simulink library "thc"  (R2021b)
settings: Solver=VariableStepAuto  StartTime=0.0  StopTime=10.0  RelTol=1e-3
undefined symbols (not defined in the file or in its folder): ATHC_APTCQA_X_C, ATHC_APTCQB_X_C, ATHC_dAy_X_C, ATHC_Qeq_X_kmh, ATHC_VbaseC_X_C, ATHC_VbaseC_Y_W, ATHC_VbaseD_X_C, ATHC_VbaseH_X_C, FALSE, KTHC_ACMaxMinT_sec, KTHC_aDeice_K, KTHC_AGSDefLv_K, KTHC_AGSLv1_K, KTHC_AGSLv2_K, KTHC_AGSLv3_K, KTHC_AGSLv4_K, KTHC_AGSLv5_K, KTHC_AirIntUpdateT_sec, KTHC_APTCOneZoneMax_W, KTHC_APTCPeriod_cnt, KTHC_APTCPWMEN_flg, KTHC_APTCQMaxC_W, KTHC_APTCQminC_W, KTHC_APTCQminD_W, KTHC_APTCQminRe1_W, KTHC_APTCQminRe_W, KTHC_APTCQoffT_cnt, KTHC_APTCQonT_cnt, KTHC_APTCRiLeMaxDff_W, KTHC_APTCRiLeMinDff_W, KTHC_BatInTempDef_C, KTHC_bDeice_K, KTHC_CompMaxDeice_rpm, KTHC_CompMinDeice_rpm, KTHC_CompSotxvOp_K, KTHC_CompSotxvOpLow_rpm, KTHC_CompSpdmax_rpm, KTHC_CompSpdmaxBC1_rpm, KTHC_CompSpdmaxBC_rpm, KTHC_CompSpdmid1_rpm, KTHC_CompSpdmid2_rpm, KTHC_CompSpdmid3_rpm, KTHC_CompSpdmid_rpm, KTHC_CompSpdmin_rpm, KTHC_DAPTCQ1_W, KTHC_DAPTCQ2_W, KTHC_DAPTCQ3_W, KTHC_DcChSetTemp_C, KTHC_DehumidityEN_flg, KTHC_DeiceCycTime_K, KTHC_DriveLevelWPTCBAH1_W, KTHC_DriveLevelWPTCBAH2_W, KTHC_DriveLevelWPTCBAH3_W, KTHC_DriveLevelWPTCBAH4_W, KTHC_DriveT1MinBAH_C, KTHC_DriveT2MaxBAH_C, KTHC_DriveT2MinBAH_C, KTHC_DriveT3MaxBAH_C, KTHC_DriveT3MinBAH_C, KTHC_DriveT4MaxBAH_C ... (+372)
libraries: simulink x140
(part 7 of 10)

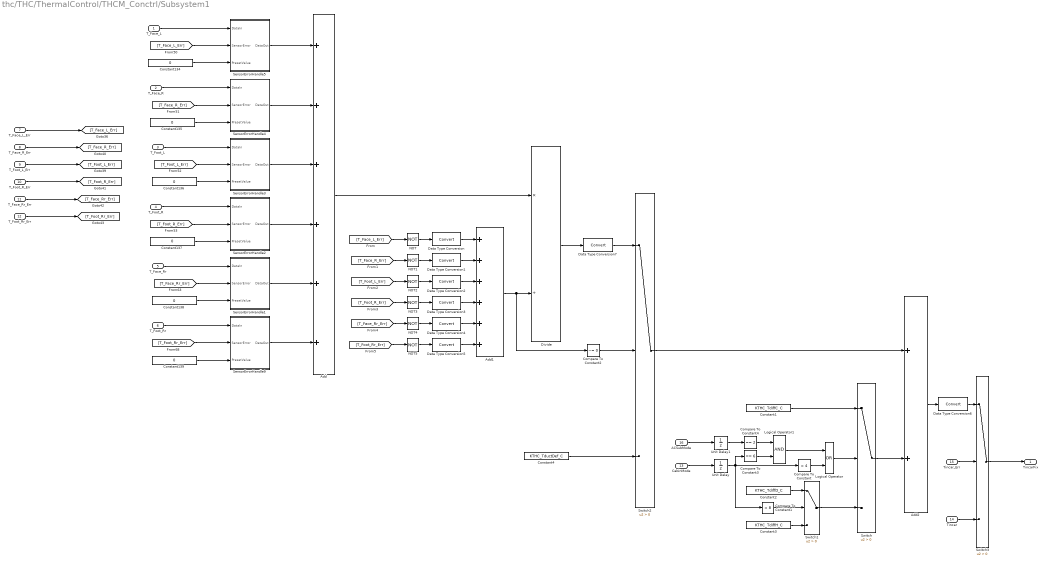
== system thc/THC/ThermalControl/THCM_Conctrl/Subsystem1 ==
  T_Face_L : Inport
  T_Face_R : Inport  Port=2
  T_Foot_L : Inport  Port=3
  T_Foot_R : Inport  Port=4
  T_Face_Rr : Inport  Port=5
  T_Foot_Rr : Inport  Port=6
  T_Face_L_Err : Inport  Port=7
  T_Face_R_Err : Inport  Port=8
  T_Foot_L_Err : Inport  Port=9
  T_Foot_R_Err : Inport  Port=10
  T_Face_Rr_Err : Inport  Port=11
  T_Foot_Rr_Err : Inport  Port=12
  CabinMode : Inport  Port=13
  Tincar : Inport  Port=14
  Tincar_Err : Inport  Port=15
  ACSubMode : Inport  Port=16
  Add : Sum  Inputs=++++++
  Add1 : Sum  Inputs=++++++
  Add2 : Sum
  Compare To Constant : simulink/Logic and Bit Operations/Compare To Constant  relop=<  const=4  OutDataTypeStr=boolean
  Compare To Constant1 : simulink/Logic and Bit Operations/Compare To Constant  relop=<  const=8  OutDataTypeStr=boolean
  Compare To Constant2 : simulink/Logic and Bit Operations/Compare To Constant  relop=~=  const=0  OutDataTypeStr=boolean
  Compare To Constant3 : simulink/Logic and Bit Operations/Compare To Constant  relop===  const=6  OutDataTypeStr=boolean
  Compare To Constant4 : simulink/Logic and Bit Operations/Compare To Constant  relop===  const=2  OutDataTypeStr=boolean
  Constant1 : Constant  Value=KTHC_TdiffC_C
  Constant{134..139} (6 alike) : Constant  Value=0
  Constant2 : Constant  Value=KTHC_TdiffD_C
  Constant3 : Constant  Value=KTHC_TdiffH_C
  Constant4 : Constant  Value=KTHC_TductDef_C
  Data Type Conversion{,1..7} (8 alike) : DataTypeConversion
  Divide : Product  Inputs=*/
  Logical Operator : Logic  Operator=OR  AllPortsSameDT=off  OutDataTypeStr=boolean
  Logical Operator1 : Logic  AllPortsSameDT=off  OutDataTypeStr=boolean
  NOT{,1..5} (6 alike) : Logic  Operator=NOT  IconShape=distinctive  AllPortsSameDT=off  OutDataTypeStr=boolean
  SensorErrorHandle1 : Subsystem
  SensorErrorHandle2 : Subsystem
  SensorErrorHandle3 : Subsystem
  SensorErrorHandle4 : Subsystem
  SensorErrorHandle5 : Subsystem
  SensorErrorHandle9 : Subsystem
  Switch{,1..3} (4 alike) : Switch  Criteria=u2 > Threshold
  Unit Delay : UnitDelay  SampleTime=-1  HasFrameUpgradeWarning=on
  Unit Delay1 : UnitDelay  SampleTime=-1  HasFrameUpgradeWarning=on
  TincarFix : Outport
  wires:
  Unit Delay1/1 -> Compare To Constant4/1
  Compare To Constant3/1 -> Logical Operator1/2
  Logical Operator1/1 -> Logical Operator/1
  Compare To Constant4/1 -> Logical Operator1/1
  ACSubMode/1 -> Unit Delay1/1
  Logical Operator/1 -> Switch/2
  Compare To Constant/1 -> Logical Operator/2
  Data Type Conversion7/1 -> Switch2/1
  Data Type Conversion6/1 -> Switch3/1
  Switch3/1 -> TincarFix/1
  Tincar/1 -> Switch3/3
  Add2/1 -> Data Type Conversion6/1
  Tincar_Err/1 -> Switch3/2
  Switch/1 -> Add2/2
  Switch2/1 -> Add2/1
  Constant4/1 -> Switch2/3
  Divide/1 -> Data Type Conversion7/1
  Compare To Constant2/1 -> Switch2/2
  Constant3/1 -> Switch1/3
  Constant2/1 -> Switch1/1
  Constant1/1 -> Switch/1
  Compare To Constant1/1 -> Switch1/2
  Switch1/1 -> Switch/3
  Unit Delay/1 -> Compare To Constant/1, Compare To Constant1/1, Compare To Constant3/1
  CabinMode/1 -> Unit Delay/1
  Add1/1 -> Divide/2, Compare To Constant2/1
  Add/1 -> Divide/1
  NOT5/1 -> Data Type Conversion5/1
  [T_Foot_Rr_Err] -> NOT5/1
  Data Type Conversion5/1 -> Add1/6
  Data Type Conversion4/1 -> Add1/5
  [T_Face_Rr_Err] -> NOT4/1
  NOT4/1 -> Data Type Conversion4/1
  NOT3/1 -> Data Type Conversion3/1
  [T_Foot_R_Err] -> NOT3/1
  Data Type Conversion3/1 -> Add1/4
  Data Type Conversion2/1 -> Add1/3
  [T_Foot_L_Err] -> NOT2/1
  NOT2/1 -> Data Type Conversion2/1
  Data Type Conversion1/1 -> Add1/2
  NOT1/1 -> Data Type Conversion1/1
  [T_Face_R_Err] -> NOT1/1
  [T_Face_L_Err] -> NOT/1
  NOT/1 -> Data Type Conversion/1
  Data Type Conversion/1 -> Add1/1
  SensorErrorHandle4/1(DataOut) -> Add/2
  SensorErrorHandle3/1(DataOut) -> Add/3
  SensorErrorHandle1/1(DataOut) -> Add/5
  SensorErrorHandle2/1(DataOut) -> Add/4
  SensorErrorHandle9/1(DataOut) -> Add/6
  SensorErrorHandle5/1(DataOut) -> Add/1
  Constant139/1 -> SensorErrorHandle9/3(PresetValue)
  [T_Foot_Rr_Err] -> SensorErrorHandle9/2(SensorError)
  Constant138/1 -> SensorErrorHandle1/3(PresetValue)
  [T_Face_Rr_Err] -> SensorErrorHandle1/2(SensorError)
  T_Face_L/1 -> SensorErrorHandle5/1(DataIn)
  Constant134/1 -> SensorErrorHandle5/3(PresetValue)
  [T_Face_L_Err] -> SensorErrorHandle5/2(SensorError)
  Constant137/1 -> SensorErrorHandle2/3(PresetValue)
  [T_Foot_R_Err] -> SensorErrorHandle2/2(SensorError)
  Constant136/1 -> SensorErrorHandle3/3(PresetValue)
  [T_Foot_L_Err] -> SensorErrorHandle3/2(SensorError)
  Constant135/1 -> SensorErrorHandle4/3(PresetValue)
  [T_Face_R_Err] -> SensorErrorHandle4/2(SensorError)
  T_Face_L_Err/1 -> [T_Face_L_Err]
  T_Face_Rr_Err/1 -> [T_Face_Rr_Err]
  T_Foot_Rr_Err/1 -> [T_Foot_Rr_Err]
  T_Foot_Rr/1 -> SensorErrorHandle9/1(DataIn)
  T_Face_Rr/1 -> SensorErrorHandle1/1(DataIn)
  T_Face_R_Err/1 -> [T_Face_R_Err]
  T_Foot_L/1 -> SensorErrorHandle3/1(DataIn)
  T_Foot_R/1 -> SensorErrorHandle2/1(DataIn)
  T_Foot_R_Err/1 -> [T_Foot_R_Err]
  T_Face_R/1 -> SensorErrorHandle4/1(DataIn)
  T_Foot_L_Err/1 -> [T_Foot_L_Err]

== system thc/THC/ThermalControl/THCM_Conctrl/Subsystem2 ==
  Motor_In_Temp : Inport
  Motor_In_Temp_Err : Inport  Port=2
  TBMax : Inport  Port=3
  Compare To Constant : simulink/Logic and Bit Operations/Compare To Constant  relop=>  const=20  OutDataTypeStr=boolean
  Constant1 : Constant  Value=KTHC_MotorInTempDefL_C
  Constant140 : Constant  Value=KTHC_MotorInTempDefH_C
  SensorErrorHandle9 : Subsystem
  Switch : Switch  Criteria=u2 > Threshold
  Motor_In_TempFix : Outport
  wires:
  SensorErrorHandle9/1(DataOut) -> Motor_In_TempFix/1
  Switch/1 -> SensorErrorHandle9/3(PresetValue)
  Motor_In_Temp_Err/1 -> SensorErrorHandle9/2(SensorError)
  Motor_In_Temp/1 -> SensorErrorHandle9/1(DataIn)
  Constant1/1 -> Switch/3
  Constant140/1 -> Switch/1
  Compare To Constant/1 -> Switch/2
  TBMax/1 -> Compare To Constant/1

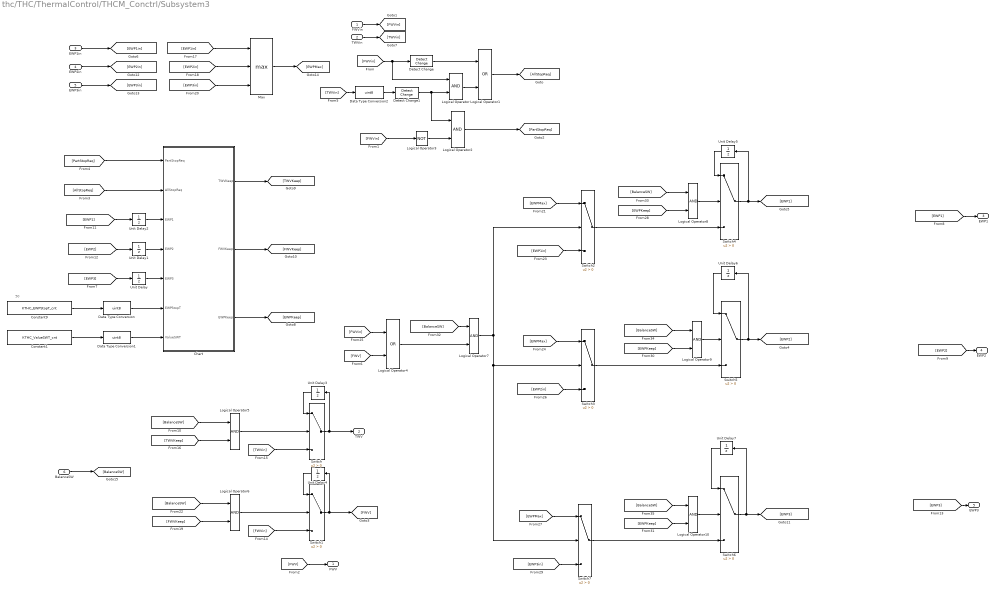
== system thc/THC/ThermalControl/THCM_Conctrl/Subsystem3 ==
  note: 50
  FWVin : Inport
  TWVin : Inport  Port=2
  EWP1in : Inport  Port=3
  EWP2in : Inport  Port=4
  EWP3in : Inport  Port=5
  BalanceSW : Inport  Port=6
  Chart : Stateflow chart  TreatAsAtomicUnit=on
  Constant1 : Constant  Value=KTHC_ValueSWT_cnt
  Constant9 : Constant  Value=KTHC_EWPStopT_cnt
  Data Type Conversion : DataTypeConversion  OutDataTypeStr=uint8
  Data Type Conversion1 : DataTypeConversion  OutDataTypeStr=uint8
  Data Type Conversion2 : DataTypeConversion  OutDataTypeStr=uint8
  Detect Change : simulink/Logic and Bit Operations/Detect Change  vinit=0  OutDataTypeStr=boolean
  Detect Change1 : simulink/Logic and Bit Operations/Detect Change  vinit=0  OutDataTypeStr=boolean
  Logical Operator{,2,5..10} (8 alike) : Logic  AllPortsSameDT=off  OutDataTypeStr=boolean
  Logical Operator1 : Logic  Operator=OR  AllPortsSameDT=off  OutDataTypeStr=boolean
  Logical Operator3 : Logic  Operator=NOT  AllPortsSameDT=off  OutDataTypeStr=boolean
  Logical Operator4 : Logic  Operator=OR  AllPortsSameDT=off  OutDataTypeStr=boolean
  Max : MinMax  Function=max  Inputs=3
  Switch{,1..7} (8 alike) : Switch  Criteria=u2 > Threshold
  Unit Delay{,1..7} (8 alike) : UnitDelay  SampleTime=-1  HasFrameUpgradeWarning=on
  FWV : Outport
  TWV : Outport  Port=2
  EWP1 : Outport  Port=3
  EWP2 : Outport  Port=4
  EWP3 : Outport  Port=5
  wires:
  [EWP2in] -> Max/2
  [FWVin] -> Switch1/3
  Switch1/1 -> Unit Delay4/1, [FWV]
  Unit Delay4/1 -> Switch1/1
  [FWVin] -> Detect Change/1, Logical Operator/1
  [EWPMax] -> Switch7/1
  [EWP3in] -> Switch7/3
  [EWP1] -> EWP1/1
  [EWPMax] -> Switch3/1
  Unit Delay3/1 -> Switch/1
  [EWP1in] -> Max/1
  Constant9/1 -> Data Type Conversion/1
  TWVin/1 -> [TWVin]
  Logical Operator1/1 -> [AllStopReq]
  Chart/2(FWVKeep) -> [FWVKeep]
  Logical Operator7/1 -> Switch7/2, Switch3/2, Switch2/2
  Unit Delay1/1 -> Chart/4(EWP2)
  [EWP3] -> EWP3/1
  [EWP1in] -> Switch2/3
  Max/1 -> [EWPMax]
  FWVin/1 -> [FWVin]
  [EWP3in] -> Max/3
  [EWP2] -> EWP2/1
  [EWPMax] -> Switch2/1
  Logical Operator2/1 -> [PartStopReq]
  [EWP2] -> Unit Delay1/1
  Switch2/1 -> Switch4/3
  Logical Operator/1 -> Logical Operator1/2
  [TWVin] -> Switch/3
  [EWP2in] -> Switch3/3
  Unit Delay2/1 -> Chart/3(EWP1)
  Unit Delay/1 -> Chart/5(EWP3)
  [FWVin] -> Logical Operator3/1
  Logical Operator3/1 -> Logical Operator2/2
  Data Type Conversion/1 -> Chart/6(EWPStopT)
  Detect Change/1 -> Logical Operator1/1
  [EWP3] -> Unit Delay/1
  Chart/1(TWVKeep) -> [TWVKeep]
  Switch/1 -> TWV/1, Unit Delay3/1
  [EWP1] -> Unit Delay2/1
  [FWV] -> FWV/1
  [FWVin] -> Logical Operator4/1
  [FWV] -> Logical Operator4/2
  [PartStopReq] -> Chart/1(PartStopReq)
  [AllStopReq] -> Chart/2(AllStopReq)
  EWP1in/1 -> [EWP1in]
  EWP2in/1 -> [EWP2in]
  EWP3in/1 -> [EWP3in]
  Constant1/1 -> Data Type Conversion1/1
  Data Type Conversion1/1 -> Chart/7(ValueSWT)
  Chart/3(EWPKeep) -> [EWPKeep]
  Unit Delay5/1 -> Switch4/1
  Switch4/1 -> Unit Delay5/1, [EWP1]
  Switch5/1 -> [EWP2], Unit Delay6/1
  Unit Delay6/1 -> Switch5/1
  Switch3/1 -> Switch5/3
  Switch7/1 -> Switch6/3
  Unit Delay7/1 -> Switch6/1
  Switch6/1 -> [EWP3], Unit Delay7/1
  BalanceSW/1 -> [BalanceSW]
  Logical Operator5/1 -> Switch/2
  [BalanceSW] -> Logical Operator5/1
  [TWVKeep] -> Logical Operator5/2
  Logical Operator6/1 -> Switch1/2
  [FWVKeep] -> Logical Operator6/2
  [BalanceSW] -> Logical Operator6/1
  Logical Operator4/1 -> Logical Operator7/2
  [BalanceSW] -> Logical Operator7/1
  Logical Operator8/1 -> Switch4/2
  [EWPKeep] -> Logical Operator8/2
  [BalanceSW] -> Logical Operator8/1
  Logical Operator9/1 -> Switch5/2
  [EWPKeep] -> Logical Operator9/2
  [BalanceSW] -> Logical Operator9/1
  Logical Operator10/1 -> Switch6/2
  [EWPKeep] -> Logical Operator10/2
  [BalanceSW] -> Logical Operator10/1
  Detect Change1/1 -> Logical Operator2/1, Logical Operator/2
  [TWVin] -> Data Type Conversion2/1
  Data Type Conversion2/1 -> Detect Change1/1

== system thc/THC/ThermalControl/THCM_Conctrl/Subsystem4 ==
  sigSetTempZon1St : Inport
  Tamb : Inport  Port=2
  Add1 : Sum
  Add2 : Sum  Inputs=+-
  Constant : Constant  Value=0.5
  Constant1 : Constant  Value=0.5
  Constant2 : Constant
  Constant3 : Constant  Value=0
  Data Type Conversion : DataTypeConversion  OutDataTypeStr=single
  Data Type Conversion1 : DataTypeConversion  OutDataTypeStr=single
  Data Type Conversion2 : DataTypeConversion  OutDataTypeStr=boolean
  Data Type Conversion3 : DataTypeConversion  OutDataTypeStr=boolean
  Relational Operator : RelationalOperator  Operator=<=  OutDataTypeStr=boolean  RndMeth=Simplest
  Relational Operator1 : RelationalOperator  Operator=>  OutDataTypeStr=boolean  RndMeth=Simplest
  Switch : Switch  Criteria=u2 > Threshold
  Switch1 : Switch  Criteria=u2 > Threshold
  Unit Delay : UnitDelay  SampleTime=-1  HasFrameUpgradeWarning=on
  HeatReq : Outport
  wires:
  [sigSetTempZon1St] -> Add1/1
  Constant/1 -> Data Type Conversion/1
  Data Type Conversion/1 -> Add1/2
  Data Type Conversion1/1 -> Add2/2
  Constant1/1 -> Data Type Conversion1/1
  [sigSetTempZon1St] -> Add2/1
  Tamb/1 -> [Tamb]
  [Tamb] -> Relational Operator/1
  Add2/1 -> Relational Operator/2
  Relational Operator/1 -> Switch/2
  Constant2/1 -> Data Type Conversion2/1
  Data Type Conversion2/1 -> Switch/1
  [Tamb] -> Relational Operator1/1
  Add1/1 -> Relational Operator1/2
  Relational Operator1/1 -> Switch1/2
  Constant3/1 -> Data Type Conversion3/1
  Data Type Conversion3/1 -> Switch1/1
  Switch1/1 -> Switch/3
  Unit Delay/1 -> Switch1/3
  Switch/1 -> HeatReq/1, Unit Delay/1
  sigSetTempZon1St/1 -> [sigSetTempZon1St]

== system thc/THC/ThermalControl/THCM_Conctrl/WPTC ==
  WPTC : Inport
  EWP3_Err : Inport  Port=2
  PresetValue : Inport  Port=3
  Constant : Constant  Value=KTHC_ErrHandleEN_flg
  Logical Operator : Logic  AllPortsSameDT=off  OutDataTypeStr=boolean
  Switch : Switch  Criteria=u2 > Threshold
  DataOut : Outport
  wires:
  Logical Operator/1 -> Switch/2
  EWP3_Err/1 -> Logical Operator/1
  Constant/1 -> Logical Operator/2
  PresetValue/1 -> Switch/1
  WPTC/1 -> Switch/3
  Switch/1 -> DataOut/1

== system thc/THC/ThermalControl/THCM_Conctrl/APTC/APTCPIControl ==
  x : Inport
  Reset : Inport  Port=2
  CtrlReset : Inport  Port=3
  VTHC_KpAPTC_K : Inport  Port=4
  VTHC_KiAPTC_K : Inport  Port=5
  Add : Sum
  Add1 : Sum
  Constant : Constant  Value=0
  Equal : RelationalOperator  Operator=~=  OutDataTypeStr=boolean  RndMeth=Simplest
  Logical Operator : Logic  Operator=OR  AllPortsSameDT=off  OutDataTypeStr=boolean
  Product : Product
  Product1 : Product
  Saturation : Saturate  UpperLimit=1  LowerLimit=0
  Switch : Switch  Criteria=u2 > Threshold
  Ts : Gain  Gain=0.1
  Unit Delay : UnitDelay  SampleTime=-1  HasFrameUpgradeWarning=on
  Unit Delay1 : UnitDelay  SampleTime=-1  HasFrameUpgradeWarning=on
  VTHC_APTCP_K : Outport
  VTHC_APTCI_K : Outport  Port=2
  VTHC_APTCU_K : Outport  Port=3
  wires:
  Logical Operator/1 -> Switch/2
  CtrlReset/1 -> Logical Operator/2
  Ts/1 -> Add1/1  "VTHC_APTCI_K"
  Product1/1 -> Ts/1
  Add1/1 -> Unit Delay1/1
  x/1 -> Product1/2, Product/2
  Saturation/1 -> Switch/3
  VTHC_KiAPTC_K/1 -> Product1/1
  VTHC_KpAPTC_K/1 -> Product/1
  Reset/1 -> Equal/1, Unit Delay/1
  Unit Delay1/1 -> Saturation/1
  Switch/1 -> Add1/2, Add/2, VTHC_APTCI_K/1  "VTHC_APTCI_K"
  Add/1 -> VTHC_APTCU_K/1
  Product/1 -> Add/1, VTHC_APTCP_K/1  "VTHC_APTCP_K"
  Constant/1 -> Switch/1
  Equal/1 -> Logical Operator/1
  Unit Delay/1 -> Equal/2

== system thc/THC/ThermalControl/THCM_Conctrl/APTC/APTCPWMControl ==
  Win : Inport
  Chart : Stateflow chart  TreatAsAtomicUnit=on
  Constant : Constant  Value=KTHC_APTCPeriod_cnt
  Constant1 : Constant  Value=KTHC_APTCQminC_W
  Constant43 : Constant  Value=KTHC_APTCPWMEN_flg
  Data Type Conversion : DataTypeConversion  OutDataTypeStr=uint16
  Data Type Conversion1 : DataTypeConversion  OutDataTypeStr=uint16
  Data Type Conversion2 : DataTypeConversion  OutDataTypeStr=uint16
  Out1 : Outport
  wires:
  Data Type Conversion/1 -> Chart/1(Win)
  Constant1/1 -> Data Type Conversion2/1
  Constant/1 -> Data Type Conversion1/1
  Data Type Conversion2/1 -> Chart/3(Wmin)
  Data Type Conversion1/1 -> Chart/2(Tp)
  Chart/1(Wout) -> Out1/1  "Wout"
  Win/1 -> Data Type Conversion/1  "Win"
  Constant43/1 -> Chart/4(KTHC_APTCPWMEN_flg)

== system thc/THC/ThermalControl/THCM_Conctrl/APTC/APTCPWMControl1 ==
  Win : Inport
  Chart : Stateflow chart  TreatAsAtomicUnit=on
  Constant : Constant  Value=KTHC_APTCPeriod_cnt
  Constant1 : Constant  Value=KTHC_APTCQminC_W
  Constant43 : Constant  Value=KTHC_APTCPWMEN_flg
  Data Type Conversion : DataTypeConversion  OutDataTypeStr=uint16
  Data Type Conversion1 : DataTypeConversion  OutDataTypeStr=uint16
  Data Type Conversion2 : DataTypeConversion  OutDataTypeStr=uint16
  Out1 : Outport
  wires:
  Constant43/1 -> Chart/4(KTHC_APTCPWMEN_flg)
  Win/1 -> Data Type Conversion/1  "Win"
  Chart/1(Wout) -> Out1/1  "Wout"
  Data Type Conversion1/1 -> Chart/2(Tp)
  Data Type Conversion2/1 -> Chart/3(Wmin)
  Constant/1 -> Data Type Conversion1/1
  Constant1/1 -> Data Type Conversion2/1
  Data Type Conversion/1 -> Chart/1(Win)

== system thc/THC/ThermalControl/THCM_Conctrl/APTC/APTCPWMControl2 ==
  Win : Inport
  Chart : Stateflow chart  TreatAsAtomicUnit=on
  Constant : Constant  Value=KTHC_APTCPeriod_cnt
  Constant1 : Constant  Value=KTHC_APTCQminC_W
  Constant43 : Constant  Value=KTHC_APTCPWMEN_flg
  Data Type Conversion : DataTypeConversion  OutDataTypeStr=uint16
  Data Type Conversion1 : DataTypeConversion  OutDataTypeStr=uint16
  Data Type Conversion2 : DataTypeConversion  OutDataTypeStr=uint16
  Out1 : Outport
  wires:
  Data Type Conversion/1 -> Chart/1(Win)
  Constant1/1 -> Data Type Conversion2/1
  Constant/1 -> Data Type Conversion1/1
  Data Type Conversion2/1 -> Chart/3(Wmin)
  Data Type Conversion1/1 -> Chart/2(Tp)
  Chart/1(Wout) -> Out1/1  "Wout"
  Win/1 -> Data Type Conversion/1  "Win"
  Constant43/1 -> Chart/4(KTHC_APTCPWMEN_flg)

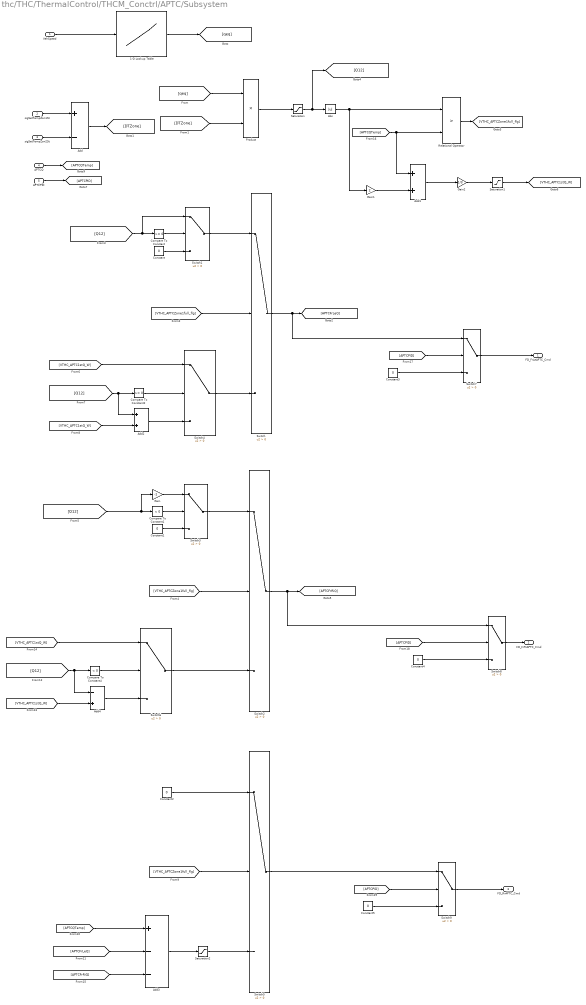
== system thc/THC/ThermalControl/THCM_Conctrl/APTC/Subsystem ==
  VehSpeed : Inport
  sigSetTempZon1St : Inport  Port=2
  sigSetTempZon2St : Inport  Port=3
  APTCQ : Inport  Port=4
  APTCPID : Inport  Port=5
  1-D Lookup Table : Lookup_n-D  NumberOfTableDimensions=1  BreakpointsForDimension1=ATHC_Qeq_X_kmh  Table=MTHC_Qeq_Y_K  InternalRulePriority=Speed  RndMeth=Simplest  InputSameDT=on
  Abs : Abs
  Add : Sum  Inputs=+-
  Add1 : Sum
  Add2 : Sum
  Add3 : Sum  Inputs=+--
  Add4 : Sum  Inputs=-+
  Compare To Constant : simulink/Logic and Bit Operations/Compare To Constant  relop=>=  const=0  OutDataTypeStr=boolean
  Compare To Constant1 : simulink/Logic and Bit Operations/Compare To Constant  relop=<  const=0  OutDataTypeStr=boolean
  Compare To Constant2 : simulink/Logic and Bit Operations/Compare To Constant  relop=>=  const=0  OutDataTypeStr=boolean
  Compare To Constant4 : simulink/Logic and Bit Operations/Compare To Constant  relop=<  const=0  OutDataTypeStr=boolean
  Constant{,1..5} (6 alike) : Constant  Value=0
  Gain : Gain  Gain=-1
  Gain1 : Gain  Gain=2
  Gain2 : Gain  Gain=1/3
  Product : Product
  Relational Operator : RelationalOperator  Operator=>  OutDataTypeStr=boolean  RndMeth=Simplest
  Saturation : Saturate  UpperLimit=KTHC_APTCRiLeMaxDff_W  LowerLimit=KTHC_APTCRiLeMinDff_W
  Saturation1 : Saturate  UpperLimit=KTHC_APTCOneZoneMax_W  LowerLimit=0
  Saturation2 : Saturate  UpperLimit=KTHC_APTCOneZoneMax_W  LowerLimit=0
  Switch{,1..9} (10 alike) : Switch  Criteria=u2 > Threshold
  FD_FrLeAPTC_Cmd : Outport
  FD_FrRiAPTC_Cmd : Outport  Port=2
  FD_RrAPTC_Cmd : Outport  Port=3
  wires:
  [APTCPID] -> Switch7/2
  APTCQ/1 -> [APTCQTemp]
  Switch9/1 -> FD_RrAPTC_Cmd/1
  Constant5/1 -> Switch9/3
  [APTCPID] -> Switch9/2
  Switch5/1 -> Switch9/1
  Switch8/1 -> FD_FrRiAPTC_Cmd/1
  Switch2/1 -> [APTCFrRiQ], Switch8/1
  [APTCPID] -> Switch8/2
  Constant4/1 -> Switch8/3
  Constant3/1 -> Switch7/3
  APTCPID/1 -> [APTCPID]
  Switch7/1 -> FD_FrLeAPTC_Cmd/1
  Saturation1/1 -> [VTHC_APTC1stQ_W]
  Constant1/1 -> Switch3/3
  Add2/1 -> Switch4/3
  Add1/1 -> Gain2/1
  [APTCQTemp] -> Relational Operator/2, Add1/1
  Product/1 -> Saturation/1
  [VTHC_APTC1stQ_W] -> Add2/2
  Gain/1 -> Switch3/1
  [VTHC_APTCZone1full_flg] -> Switch5/2
  sigSetTempZon1St/1 -> Add/1
  Compare To Constant1/1 -> Switch3/2
  [Q12] -> Compare To Constant4/1, Add4/1
  [VTHC_APTC1stQ_W] -> Switch6/1
  Switch1/1 -> Switch/1
  Compare To Constant2/1 -> Switch4/2
  Switch3/1 -> Switch2/1
  Abs/1 -> Relational Operator/1, Gain1/1
  Add/1 -> [DTZone]
  [DTZone] -> Product/2
  [Q12] -> Compare To Constant1/1, Gain/1
  [VTHC_APTCZone1full_flg] -> Switch2/2
  Add3/1 -> Saturation2/1
  Relational Operator/1 -> [VTHC_APTCZone1full_flg]
  [Q12] -> Compare To Constant/1, Switch1/1
  sigSetTempZon2St/1 -> Add/2
  [VTHC_APTCZone1full_flg] -> Switch/2
  [APTCFrLeQ] -> Add3/2
  Compare To Constant/1 -> Switch1/2
  Compare To Constant4/1 -> Switch6/2
  Constant2/1 -> Switch5/1
  Add4/1 -> Switch6/3
  [VTHC_APTC1stQ_W] -> Add4/2
  Switch/1 -> [APTCFrLeQ], Switch7/1
  Gain2/1 -> Saturation1/1
  Saturation/1 -> Abs/1, [Q12]
  Switch4/1 -> Switch/3
  Switch6/1 -> Switch2/3
  [Q12] -> Compare To Constant2/1, Add2/1
  [APTCFrRiQ] -> Add3/3
  Saturation2/1 -> Switch5/3
  Gain1/1 -> Add1/2
  1-D Lookup Table/1 -> [qeq]
  Constant/1 -> Switch1/3
  [qeq] -> Product/1
  [APTCQTemp] -> Add3/1
  VehSpeed/1 -> 1-D Lookup Table/1
  [VTHC_APTC1stQ_W] -> Switch4/1

== system thc/THC/ThermalControl/THCM_Conctrl/BlowerCtrl/BlowerPIControl ==
  x : Inport
  Reset : Inport  Port=2
  VTHC_BlowerKp_K : Inport  Port=3
  VTHC_BlowerKi_K : Inport  Port=4
  Add : Sum
  Add1 : Sum
  Constant : Constant  Value=0
  Equal : RelationalOperator  Operator=~=  OutDataTypeStr=boolean  RndMeth=Simplest
  Product : Product
  Product1 : Product
  Saturation : Saturate  UpperLimit=1  LowerLimit=0
  Switch : Switch  Criteria=u2 > Threshold
  Ts : Gain  Gain=0.1
  Unit Delay : UnitDelay  SampleTime=-1  HasFrameUpgradeWarning=on
  Unit Delay1 : UnitDelay  SampleTime=-1  HasFrameUpgradeWarning=on
  VTHC_BlowerP_K : Outport
  VTHC_BlowerI_K : Outport  Port=2
  VTHC_BlowerU_K : Outport  Port=3
  wires:
  Saturation/1 -> Switch/3
  Unit Delay1/1 -> Saturation/1
  Ts/1 -> Add1/1
  VTHC_BlowerKi_K/1 -> Product1/2
  VTHC_BlowerKp_K/1 -> Product/1
  Switch/1 -> Add/2, VTHC_BlowerI_K/1, Add1/2  "VTHC_BlowerI_K"
  Product1/1 -> Ts/1
  Add1/1 -> Unit Delay1/1
  Add/1 -> VTHC_BlowerU_K/1
  Product/1 -> Add/1, VTHC_BlowerP_K/1  "VTHC_BlowerP_K"
  x/1 -> Product1/1, Product/2
  Constant/1 -> Switch/1
  Equal/1 -> Switch/2
  Unit Delay/1 -> Equal/2
  Reset/1 -> Equal/1, Unit Delay/1

== system thc/THC/ThermalControl/THCM_Conctrl/BlowerCtrl/Enabled Subsystem1 ==
  Blowersolar : Inport
  Tamb : Inport  Port=2
  CabinMode : Inport  Port=3
  ACAuto : Inport  Port=4
  Vmanual : Inport  Port=5
  DfrstReq : Inport  Port=6
  ACSubMode : Inport  Port=7
  PwrSta : Inport  Port=8
  1-D Lookup Table : Lookup_n-D  NumberOfTableDimensions=1  BreakpointsForDimension1=ATHC_VbaseH_X_C  Table=MTHC_VbaseH_Y_K  InternalRulePriority=Speed  RndMeth=Simplest  InputSameDT=on
  1-D Lookup Table1 : Lookup_n-D  NumberOfTableDimensions=1  BreakpointsForDimension1=ATHC_VbaseD_X_C  Table=MTHC_VbaseD_Y_K  InternalRulePriority=Speed  RndMeth=Simplest  InputSameDT=on
  2-D Lookup Table1 : Lookup_n-D  BreakpointsForDimension1=ATHC_VbaseC_Y_W  BreakpointsForDimension2=ATHC_VbaseC_X_C  Table=MTHC_VbaseC_Z_K  InternalRulePriority=Speed  RndMeth=Simplest  InputSameDT=on
      settings: InputPortMap=u0,u1
  Chart2 : Stateflow chart  TreatAsAtomicUnit=on
      settings: PortSchema="{\"entries\":[{\"content\":{\"sides\":[{\"content\":{\"connectorIds\":[\"In1\",\"In2\",\"In3\",\"In4\",\"In5\",\"In6\",\"In7\",\"In8\",\"In9\",\"In10\",\"In11\",\"In12\",\"In14\",\"In13\"]},\"type\":\"ConnectorPlacement.EquallySpacedRectSide\",\"uuid\":\"7e8f7538-56f4-447a-9145-c20cc29664fa\"},{\"content\":{\"connectorIds\":[\"Out1\"],\"side\":\"RIGHT\"},\"type\":\"ConnectorPlacement.EquallySpacedRectSide\",\"uuid\":\"8e6754a2-1b4c-4aa6-81e0-e2cdf3e8c159\"},{\"content\":{\"connectorIds\":[],\"side\":\"TOP\"},\"type\":\"ConnectorPlacement.EquallySpacedRectSide\",\"uuid\":\"22019b22-c6fe-41ab-ac44-688f1d70e28d\"}]},\"type\":\"ConnectorPlacement.EquallySpacedConnector\",\"uuid\":\"3c722edc-0b93-4b6c-89cb-f70cbb5ccb6e\"}],\"packageUris\":[\"http://schema.mathworks.com/mf0/Connector/R2020b\"],\"version\":\"1.0\"}"
  Constant : Constant  Value=KTHC_VBlowerdfog_K
  Constant1 : Constant  Value=KTHC_VBlowerMin_K
  Constant2 : Constant  Value=KTHC_VBlowerMid_K
  Constant3 : Constant  Value=KTHC_VBlowerSetLow_K
  Constant4 : Constant  Value=KTHC_VBlowerDcCh_K
  VBase : Outport
  wires:
  Constant4/1 -> Chart2/13(KTHC_VBlowerDcCh_K)
  Constant3/1 -> Chart2/14(KTHC_VBlowerSetLow_K)
  Constant2/1 -> Chart2/12(KTHC_VBlowerMid_K)
  Constant1/1 -> Chart2/11(KTHC_VBlowerMin_K)
  Constant/1 -> Chart2/10(KTHC_VBlowerdfog_K)
  PwrSta/1 -> Chart2/9(PwrSta)
  1-D Lookup Table1/1 -> Chart2/6(VbaseD)  "VBaseD"
  [Tamb] -> 1-D Lookup Table1/1  "Tamb"
  ACSubMode/1 -> Chart2/2(ACSubMode)
  DfrstReq/1 -> Chart2/4(DfrstReq)
  Chart2/1(Voffset) -> VBase/1
  ACAuto/1 -> Chart2/1(ACAuto)
  CabinMode/1 -> Chart2/3(CabinMode)  "CabinMode"
  Vmanual/1 -> Chart2/8(Vmanual)
  [Tamb] -> 1-D Lookup Table/1  "Tamb"
  2-D Lookup Table1/1 -> Chart2/5(VbaseC)  "VbaseC"
  [Tamb] -> 2-D Lookup Table1/2  "Tamb"
  Blowersolar/1 -> 2-D Lookup Table1/1  "Blowersolar"
  1-D Lookup Table/1 -> Chart2/7(VbaseH)  "VBaseH"
  Tamb/1 -> [Tamb]

== system thc/THC/ThermalControl/THCM_Conctrl/CompCtrl/CompPIControl ==
  x : Inport
  Reset : Inport  Port=2
  VTHC_CompKp_K : Inport  Port=3
  VTHC_CompKi_K : Inport  Port=4
  Add : Sum
  Add1 : Sum
  Compare To Constant : simulink/Logic and Bit Operations/Compare To Constant  relop=>  const=0  OutDataTypeStr=boolean
  Constant : Constant  Value=0
  Equal : RelationalOperator  Operator=~=  OutDataTypeStr=boolean  RndMeth=Simplest
  Logical Operator : Logic  AllPortsSameDT=off  OutDataTypeStr=boolean
  Product : Product
  Product1 : Product
  Switch : Switch  Criteria=u2 > Threshold
  Ts : Gain  Gain=0.1
  Unit Delay : UnitDelay  SampleTime=-1  HasFrameUpgradeWarning=on
  Unit Delay1 : UnitDelay  SampleTime=-1  HasFrameUpgradeWarning=on
  VTHC_CompP_K : Outport
  VTHC_CompI_K : Outport  Port=2
  VTHC_CompU_K : Outport  Port=3
  wires:
  VTHC_CompKi_K/1 -> Product1/1
  VTHC_CompKp_K/1 -> Product/1
  Compare To Constant/1 -> Logical Operator/2
  Unit Delay1/1 -> Switch/3
  Ts/1 -> Add/2, VTHC_CompI_K/1  "VTHC_CompI_K"
  Product1/1 -> Ts/1
  Switch/1 -> Product1/2, Add1/2
  Add1/1 -> Unit Delay1/1
  Add/1 -> VTHC_CompU_K/1
  Product/1 -> Add/1, VTHC_CompP_K/1  "VTHC_CompP_K"
  x/1 -> Add1/1, Product/2
  Constant/1 -> Switch/1
  Logical Operator/1 -> Switch/2
  Equal/1 -> Logical Operator/1
  Unit Delay/1 -> Equal/2
  Reset/1 -> Equal/1, Unit Delay/1, Compare To Constant/1

== system thc/THC/ThermalControl/THCM_Conctrl/CompCtrl/DeltaUReset ==
  DeltaUin : Inport
  CompPID : Inport  Port=2
  TSetpoint : Inport  Port=3
  Constant1 : Constant  Value=0
  Data Type Conversion : DataTypeConversion  OutDataTypeStr=uint32
  Gain : Gain  Gain=1000
  Logical Operator : Logic  AllPortsSameDT=off  OutDataTypeStr=boolean
  Relational Operator : RelationalOperator  Operator===  OutDataTypeStr=boolean  RndMeth=Simplest
  Relational Operator1 : RelationalOperator  Operator===  OutDataTypeStr=boolean  RndMeth=Simplest
  Switch2 : Switch  Criteria=u2 > Threshold
  Unit Delay : UnitDelay  SampleTime=-1  HasFrameUpgradeWarning=on
  Unit Delay1 : UnitDelay  SampleTime=-1  HasFrameUpgradeWarning=on
  DeltaU : Outport
  wires:
  Data Type Conversion/1 -> Relational Operator/2, Unit Delay1/1
  TSetpoint/1 -> Gain/1
  Relational Operator1/1 -> Logical Operator/1
  Relational Operator/1 -> Logical Operator/2
  Unit Delay1/1 -> Relational Operator/1
  Gain/1 -> Data Type Conversion/1
  Logical Operator/1 -> Switch2/2
  Unit Delay/1 -> Relational Operator1/1
  Constant1/1 -> Switch2/3
  DeltaUin/1 -> Switch2/1
  Switch2/1 -> DeltaU/1
  CompPID/1 -> Unit Delay/1, Relational Operator1/2

== system thc/THC/ThermalControl/THCM_Conctrl/CompCtrl/Enabled Subsystem ==
  sigSetTempZon1StC : Inport
  Tincar : Inport  Port=2
  Tamb : Inport  Port=3
  VINP_SmartEcoModeSW_flg : Inport  Port=4
  Enable : EnablePort
  Chart : Stateflow chart  TreatAsAtomicUnit=on
  Constant : Constant  Value=KTHC_DTymin1_K
  Constant1 : Constant  Value=KTHC_Tambmin_C
  Constant10 : Constant  Value=KTHC_T4Maxamb_C
  Constant11 : Constant  Value=KTHC_T2Minamb_C
  Constant12 : Constant  Value=KTHC_T3Minamb_C
  Constant13 : Constant  Value=KTHC_T4Minamb_C
  Constant14 : Constant  Value=KTHC_T5Minamb_C
  Constant3 : Constant  Value=KTHC_DTymin2_K
  Constant4 : Constant  Value=KTHC_DTymin3_K
  Constant5 : Constant  Value=KTHC_DTymin4_K
  Constant6 : Constant  Value=KTHC_DTymin5_K
  Constant7 : Constant  Value=KTHC_T1Maxamb_C
  Constant8 : Constant  Value=KTHC_T2Maxamb_C
  Constant9 : Constant  Value=KTHC_T3Maxamb_C
  Product : Product
  Relational Operator1 : RelationalOperator  OutDataTypeStr=boolean  RndMeth=Simplest
  Sum : Sum  Inputs=|+-
  Switch : Switch  Criteria=u2 > Threshold
  Switch1 : Switch  Criteria=u2 > Threshold
  TincarCe : Outport
  TincarCset : Outport  Port=2
  wires:
  VINP_SmartEcoModeSW_flg/1 -> Switch1/2
  Product/1 -> Switch1/1
  [Tamb] -> Relational Operator1/1
  [DTymin] -> Product/1
  Chart/1(DTymin) -> [DTymin]
  Constant14/1 -> Chart/14(KTHC_T5Minamb_C)
  Constant13/1 -> Chart/13(KTHC_T4Minamb_C)
  Constant12/1 -> Chart/12(KTHC_T3Minamb_C)
  Constant11/1 -> Chart/11(KTHC_T2Minamb_C)
  Constant10/1 -> Chart/10(KTHC_T4Maxamb_C)
  Constant9/1 -> Chart/9(KTHC_T3Maxamb_C)
  Constant8/1 -> Chart/8(KTHC_T2Maxamb_C)
  Constant7/1 -> Chart/7(KTHC_T1Maxamb_C)
  Constant6/1 -> Chart/6(KTHC_DTymin5_K)
  Constant5/1 -> Chart/5(KTHC_DTymin4_K)
  Constant4/1 -> Chart/4(KTHC_DTymin3_K)
  Constant3/1 -> Chart/3(KTHC_DTymin2_K)
  Constant/1 -> Chart/2(KTHC_DTymin1_K)
  [Tamb] -> Chart/1(Tamb)
  Tamb/1 -> [Tamb]
  Relational Operator1/1 -> Switch/2
  Constant1/1 -> Relational Operator1/2
  Sum/1 -> Switch1/3, Product/2, Switch/3
  Switch/1 -> TincarCe/1
  Switch1/1 -> Switch/1
  Tincar/1 -> Sum/2
  sigSetTempZon1StC/1 -> TincarCset/1, Sum/1  "sigSetTempZon1StC"

== system thc/THC/ThermalControl/THCM_Conctrl/CompCtrl/Enabled Subsystem1 ==
  TBMax : Inport
  Bat_In_Temp : Inport  Port=2
  Enable : EnablePort
  Chart : Stateflow chart  TreatAsAtomicUnit=on
  Constant : Constant  Value=KTHC_T1MaxBC_C
  Constant1 : Constant  Value=KTHC_T1winSetpointBC_C
  Constant10 : Constant  Value=KTHC_T3MinBC_C
  Constant11 : Constant  Value=KTHC_T3MaxBC_C
  Constant12 : Constant  Value=KTHC_T4MinBC_C
  Constant14 : Constant  Value=KTHC_T4MaxBC_C
  Constant15 : Constant  Value=KTHC_T5MinBC_C
  Constant2 : Constant  Value=KTHC_T2winSetpointBC_C
  Constant3 : Constant  Value=KTHC_T3winSetpointBC_C
  Constant4 : Constant  Value=KTHC_T4winSetpointBC_C
  Constant5 : Constant  Value=KTHC_T5winSetpointBC_C
  Constant8 : Constant  Value=KTHC_T2MinBC_C
  Constant9 : Constant  Value=KTHC_T2MaxBC_C
  Sum : Sum  Inputs=|+-
  BatIne : Outport
  BatInset : Outport  Port=2
  wires:
  Constant5/1 -> Chart/14(KTHC_T5winSetpointBC_C)
  Constant4/1 -> Chart/13(KTHC_T4winSetpointBC_C)
  Constant3/1 -> Chart/12(KTHC_T3winSetpointBC_C)
  Constant2/1 -> Chart/11(KTHC_T2winSetpointBC_C)
  Constant1/1 -> Chart/10(KTHC_T1winSetpointBC_C)
  Constant15/1 -> Chart/9(KTHC_T5MinBC_C)
  Constant14/1 -> Chart/8(KTHC_T4MaxBC_C)
  Constant12/1 -> Chart/7(KTHC_T4MinBC_C)
  Constant11/1 -> Chart/6(KTHC_T3MaxBC_C)
  Constant10/1 -> Chart/5(KTHC_T3MinBC_C)
  Constant9/1 -> Chart/4(KTHC_T2MaxBC_C)
  Constant8/1 -> Chart/3(KTHC_T2MinBC_C)
  Constant/1 -> Chart/2(KTHC_T1MaxBC_C)
  Sum/1 -> BatIne/1
  Bat_In_Temp/1 -> Sum/2
  Chart/1(Bat_In_TempSetPoint) -> Sum/1, BatInset/1  "Bat_In_TempSetPoint"
  TBMax/1 -> Chart/1(TBMax)

== system thc/THC/ThermalControl/THCM_Conctrl/CompCtrl/Enabled Subsystem2 ==
  sigSetTempZon1St : Inport
  Tincar : Inport  Port=2
  Enable : EnablePort
  Sum : Sum  Inputs=|+-
  Tincare : Outport
  Tincarset : Outport  Port=2
  wires:
  Tincar/1 -> Sum/2
  Sum/1 -> Tincare/1
  sigSetTempZon1St/1 -> Sum/1, Tincarset/1

== system thc/THC/ThermalControl/THCM_Conctrl/CompCtrl/Enabled Subsystem3 ==
  PT_Low_P2 : Inport
  PT_ Low_P2Setpoint : Inport  Port=2
  Enable : EnablePort
  Sum : Sum  Inputs=|+-
  PTLowP2e : Outport
  wires:
  Sum/1 -> PTLowP2e/1
  PT_ Low_P2Setpoint/1 -> Sum/1
  PT_Low_P2/1 -> Sum/2

== system thc/THC/ThermalControl/THCM_Conctrl/CompCtrl/Enabled Subsystem4 ==
  PT_High_P : Inport
  PT_High_PSetpoint : Inport  Port=2
  Enable : EnablePort
  Sum : Sum  Inputs=|+-
  PT_High_Pe : Outport
  wires:
  PT_High_P/1 -> Sum/2
  PT_High_PSetpoint/1 -> Sum/1
  Sum/1 -> PT_High_Pe/1

== system thc/THC/ThermalControl/THCM_Conctrl/CompCtrl/Enabled Subsystem5 ==
  PT_Low_P1 : Inport
  PT_Low_P1Setpoint : Inport  Port=2
  Enable : EnablePort
  Sum : Sum  Inputs=|+-
  PT_Low_Pe : Outport
  wires:
  Sum/1 -> PT_Low_Pe/1
  PT_Low_P1Setpoint/1 -> Sum/1
  PT_Low_P1/1 -> Sum/2

== system thc/THC/ThermalControl/THCM_Conctrl/EXV1Ctrl/EXV1PIControl ==
  x : Inport
  Reset : Inport  Port=2
  VTHC_KpEXV1SH_K : Inport  Port=3
  VTHC_KiEXV1SH_K : Inport  Port=4
  Add : Sum
  Add1 : Sum
  Constant : Constant  Value=0
  Product : Product
  Product1 : Product
  Saturation : Saturate  UpperLimit=0.1  LowerLimit=-0.9
  Switch : Switch  Criteria=u2 > Threshold
  Ts : Gain  Gain=0.1
  Unit Delay1 : UnitDelay  SampleTime=-1  HasFrameUpgradeWarning=on
  VTHC_EXV1P_K : Outport
  VTHC_EXV1I_K : Outport  Port=2
  VTHC_EXV1U_K : Outport  Port=3
  wires:
  Ts/1 -> Add1/1  "VTHC_EXV1I_K"
  Saturation/1 -> Switch/3
  Reset/1 -> Switch/2
  VTHC_KiEXV1SH_K/1 -> Product1/2
  VTHC_KpEXV1SH_K/1 -> Product/1
  Unit Delay1/1 -> Saturation/1
  Switch/1 -> Add1/2, Add/2, VTHC_EXV1I_K/1  "VTHC_EXV1I_K"
  Product1/1 -> Ts/1
  Add1/1 -> Unit Delay1/1
  Add/1 -> VTHC_EXV1U_K/1
  Product/1 -> Add/1, VTHC_EXV1P_K/1  "VTHC_EXV1P_K"
  x/1 -> Product1/1, Product/2
  Constant/1 -> Switch/1

== system thc/THC/ThermalControl/THCM_Conctrl/EXV2Ctrl/EXV2PIControl ==
  x : Inport
  Reset : Inport  Port=2
  VTHC_KpEXV2_K : Inport  Port=3
  VTHC_KiEXV2_K : Inport  Port=4
  Add : Sum
  Add1 : Sum
  Constant : Constant  Value=0
  Equal : RelationalOperator  Operator=~=  OutDataTypeStr=boolean  RndMeth=Simplest
  Product : Product
  Product1 : Product
  Saturation : Saturate  UpperLimit=0.1  LowerLimit=-0.9
  Switch : Switch  Criteria=u2 > Threshold
  Ts : Gain  Gain=0.1
  Unit Delay : UnitDelay  SampleTime=-1  HasFrameUpgradeWarning=on
  Unit Delay1 : UnitDelay  SampleTime=-1  HasFrameUpgradeWarning=on
  VTHC_EXV2P_K : Outport
  VTHC_EXV2I_K : Outport  Port=2
  VTHC_EXV2U_K : Outport  Port=3
  wires:
  Saturation/1 -> Switch/3
  Unit Delay1/1 -> Saturation/1
  Ts/1 -> Add1/1
  VTHC_KiEXV2_K/1 -> Product1/2
  VTHC_KpEXV2_K/1 -> Product/1
  Reset/1 -> Equal/1, Unit Delay/1
  Switch/1 -> Add1/2, Add/2, VTHC_EXV2I_K/1  "VTHC_EXV2I_K"
  Product1/1 -> Ts/1
  Add1/1 -> Unit Delay1/1
  Add/1 -> VTHC_EXV2U_K/1
  Product/1 -> Add/1, VTHC_EXV2P_K/1  "VTHC_EXV2P_K"
  x/1 -> Product/2, Product1/1
  Constant/1 -> Switch/1
  Equal/1 -> Switch/2
  Unit Delay/1 -> Equal/2

== system thc/THC/ThermalControl/THCM_Conctrl/Subsystem1/SensorErrorHandle1 ==
  DataIn : Inport
  SensorError : Inport  Port=2
  PresetValue : Inport  Port=3
  Constant : Constant  Value=KTHC_ErrHandleEN_flg
  Logical Operator : Logic  AllPortsSameDT=off  OutDataTypeStr=boolean
  Switch : Switch  Criteria=u2 > Threshold
  DataOut : Outport
  wires:
  Constant/1 -> Logical Operator/2
  SensorError/1 -> Logical Operator/1
  Logical Operator/1 -> Switch/2
  Switch/1 -> DataOut/1
  DataIn/1 -> Switch/3
  PresetValue/1 -> Switch/1

== system thc/THC/ThermalControl/THCM_Conctrl/Subsystem1/SensorErrorHandle2 ==
  DataIn : Inport
  SensorError : Inport  Port=2
  PresetValue : Inport  Port=3
  Constant : Constant  Value=KTHC_ErrHandleEN_flg
  Logical Operator : Logic  AllPortsSameDT=off  OutDataTypeStr=boolean
  Switch : Switch  Criteria=u2 > Threshold
  DataOut : Outport
  wires:
  PresetValue/1 -> Switch/1
  DataIn/1 -> Switch/3
  Switch/1 -> DataOut/1
  Logical Operator/1 -> Switch/2
  SensorError/1 -> Logical Operator/1
  Constant/1 -> Logical Operator/2

== system thc/THC/ThermalControl/THCM_Conctrl/Subsystem1/SensorErrorHandle3 ==
  DataIn : Inport
  SensorError : Inport  Port=2
  PresetValue : Inport  Port=3
  Constant : Constant  Value=KTHC_ErrHandleEN_flg
  Logical Operator : Logic  AllPortsSameDT=off  OutDataTypeStr=boolean
  Switch : Switch  Criteria=u2 > Threshold
  DataOut : Outport
  wires:
  Constant/1 -> Logical Operator/2
  SensorError/1 -> Logical Operator/1
  Logical Operator/1 -> Switch/2
  Switch/1 -> DataOut/1
  DataIn/1 -> Switch/3
  PresetValue/1 -> Switch/1

== system thc/THC/ThermalControl/THCM_Conctrl/Subsystem1/SensorErrorHandle4 ==
  DataIn : Inport
  SensorError : Inport  Port=2
  PresetValue : Inport  Port=3
  Constant : Constant  Value=KTHC_ErrHandleEN_flg
  Logical Operator : Logic  AllPortsSameDT=off  OutDataTypeStr=boolean
  Switch : Switch  Criteria=u2 > Threshold
  DataOut : Outport
  wires:
  PresetValue/1 -> Switch/1
  DataIn/1 -> Switch/3
  Switch/1 -> DataOut/1
  Logical Operator/1 -> Switch/2
  SensorError/1 -> Logical Operator/1
  Constant/1 -> Logical Operator/2

== system thc/THC/ThermalControl/THCM_Conctrl/Subsystem1/SensorErrorHandle5 ==
  DataIn : Inport
  SensorError : Inport  Port=2
  PresetValue : Inport  Port=3
  Constant : Constant  Value=KTHC_ErrHandleEN_flg
  Logical Operator : Logic  AllPortsSameDT=off  OutDataTypeStr=boolean
  Switch : Switch  Criteria=u2 > Threshold
  DataOut : Outport
  wires:
  Constant/1 -> Logical Operator/2
  SensorError/1 -> Logical Operator/1
  Logical Operator/1 -> Switch/2
  Switch/1 -> DataOut/1
  DataIn/1 -> Switch/3
  PresetValue/1 -> Switch/1

== system thc/THC/ThermalControl/THCM_Conctrl/Subsystem1/SensorErrorHandle9 ==
  DataIn : Inport
  SensorError : Inport  Port=2
  PresetValue : Inport  Port=3
  Constant : Constant  Value=KTHC_ErrHandleEN_flg
  Logical Operator : Logic  AllPortsSameDT=off  OutDataTypeStr=boolean
  Switch : Switch  Criteria=u2 > Threshold
  DataOut : Outport
  wires:
  PresetValue/1 -> Switch/1
  DataIn/1 -> Switch/3
  Switch/1 -> DataOut/1
  Logical Operator/1 -> Switch/2
  SensorError/1 -> Logical Operator/1
  Constant/1 -> Logical Operator/2

== system thc/THC/ThermalControl/THCM_Conctrl/Subsystem2/SensorErrorHandle9 ==
  DataIn : Inport
  SensorError : Inport  Port=2
  PresetValue : Inport  Port=3
  Constant : Constant  Value=KTHC_ErrHandleEN_flg
  Logical Operator : Logic  AllPortsSameDT=off  OutDataTypeStr=boolean
  Switch : Switch  Criteria=u2 > Threshold
  DataOut : Outport
  wires:
  PresetValue/1 -> Switch/1
  DataIn/1 -> Switch/3
  Switch/1 -> DataOut/1
  Logical Operator/1 -> Switch/2
  SensorError/1 -> Logical Operator/1
  Constant/1 -> Logical Operator/2

== stateflow chart thc/THC/ThermalControl/THCM_Conctrl/APTC/APTCPWMControl/Chart ==
  state APTC
    en:
    Wout=Win;
    du:
    Wout=Win;
  state APTCPWM
    (default) -> (junction 5) : {Tcnt=0;OnT=0;OffT=0;}
    APTCPWM -> (junction 5) [order 1]
    (junction 5) -> (junction 7) [order 1] : [Win==0]{Wout=0;}
    (junction 5) -> (junction 9) [order 2]
    (junction 7) -> (junction 11)
    (junction 9) -> (junction 11) [order 1] : [Win>Wmin]{Wout=Win;}
    (junction 9) -> (junction 54) [order 2]
    (junction 11) -> (junction 56)
    (junction 54) -> (junction 56) [order 1] : [Wout>Wmin]{Tcnt=0;Wout=0;....
        | OnT=Tp*Win/Wmin;OffT=Tp-OnT;}
    (junction 54) -> (junction 13) [order 2]
    (junction 56) -> (junction 15)
    (junction 13) -> (junction 15) [order 1] : [Wout>0&&Tcnt>=OnT]
        | {Tcnt=0;Wout=0;}
    (junction 13) -> (junction 17) [order 2]
    (junction 15) -> (junction 19)
    (junction 17) -> (junction 19) [order 1] : [Wout==0&&Tcnt>=OffT]
        | {Tcnt=0;Wout=Wmin;....
        | OnT=Tp*Win/Wmin;OffT=Tp-OnT;}
    (junction 17) -> (junction 26) [order 2]
    (junction 19) -> (junction 28)
    (junction 26) -> (junction 28)
    (junction 28) -> (junction 31) [order 2] : {Tcnt=Tcnt+1;}
    (junction 28) -> (junction 33) [order 1] : [Tcnt>Tp||(OnT==0&&OffT==0)]
        | {Tcnt=0;OnT=0;OffT=0;}
  (default) -> (junction 50)
  (junction 50) -> APTC [order 1] : [!KTHC_APTCPWMEN_flg]
  (junction 50) -> APTCPWM [order 2]
  APTCPWM -> APTC [order 1] : [!KTHC_APTCPWMEN_flg]
  APTC -> APTCPWM : [KTHC_APTCPWMEN_flg]
  data: OnT local uint16; OffT local uint16; Tcnt local uint16; Win input; Wout output uint16; Tp input uint16; Wmin input; KTHC_APTCPWMEN_flg input

== stateflow chart thc/THC/ThermalControl/THCM_Conctrl/Chart2 ==
  state FactorSolar1
    en:FactorSolar=0.88;Blowersolar=1000;
    state Low
    state Mid
    (default) -> FactorSolar1.Mid
    FactorSolar1.Mid -> FactorSolar1.Low : [Solar<950]
    FactorSolar1.Low -> FactorSolar1.Mid [order 1] : [Solar>=950]
  state FactorSolar2
    en:FactorSolar=0.90;Blowersolar=860;
    state Low
    state Mid
    state High
    (default) -> FactorSolar2.Mid
    FactorSolar2.Mid -> FactorSolar2.High [order 2] : [Solar>1000]
    FactorSolar2.Mid -> FactorSolar2.Low [order 1] : [Solar<800]
    FactorSolar2.Low -> FactorSolar2.Mid [order 1] : [Solar>=800]
    FactorSolar2.High -> FactorSolar2.Mid [order 2] : [Solar<=1000]
  state FactorSolar3
    en:FactorSolar=0.92;Blowersolar=715;
    state Low
    state Mid
    state High
    (default) -> FactorSolar3.Mid
    FactorSolar3.Mid -> FactorSolar3.High [order 2] : [Solar>850]
    FactorSolar3.Mid -> FactorSolar3.Low [order 1] : [Solar<650]
    FactorSolar3.Low -> FactorSolar3.Mid [order 1] : [Solar>=650]
    FactorSolar3.High -> FactorSolar3.Mid [order 1] : [Solar<=850]
  state FactorSolar4
    en:FactorSolar=0.94;Blowersolar=570;
    state Low
    state Mid
    state High
    (default) -> FactorSolar4.Mid
    FactorSolar4.Mid -> FactorSolar4.High [order 2] : [Solar>700]
    FactorSolar4.Mid -> FactorSolar4.Low [order 1] : [Solar<500]
    FactorSolar4.Low -> FactorSolar4.Mid [order 1] : [Solar>=500]
    FactorSolar4.High -> FactorSolar4.Mid [order 1] : [Solar<=700]
  state FactorSolar5
    en:FactorSolar=0.96;Blowersolar=430;
    state Low
    state Mid
    state High
    (default) -> FactorSolar5.Mid
    FactorSolar5.Mid -> FactorSolar5.High [order 2] : [Solar>550]
    FactorSolar5.Mid -> FactorSolar5.Low [order 1] : [Solar<350]
    FactorSolar5.Low -> FactorSolar5.Mid [order 1] : [Solar>=350]
    FactorSolar5.High -> FactorSolar5.Mid [order 1] : [Solar<=550]
  state FactorSolar6
    en:FactorSolar=0.98;Blowersolar=285;
    state Low
    state Mid
    state High
    (default) -> FactorSolar6.Mid
    FactorSolar6.Mid -> FactorSolar6.High [order 2] : [Solar>400]
    FactorSolar6.Mid -> FactorSolar6.Low [order 1] : [Solar<200]
    FactorSolar6.Low -> FactorSolar6.Mid : [Solar>=200]
    FactorSolar6.High -> FactorSolar6.Mid [order 1] : [Solar<=400]
  state FactorSolar7
    en:FactorSolar=1;Blowersolar=100;
    state Mid
    state High
    (default) -> FactorSolar7.Mid
    FactorSolar7.Mid -> FactorSolar7.High : [Solar>250]
    FactorSolar7.High -> FactorSolar7.Mid [order 1] : [Solar<=250]
  (default) -> (junction 9)
  (junction 9) -> FactorSolar1 [order 1] : [Solar>950]
  (junction 9) -> (junction 11) [order 2]
  FactorSolar1.Low -> FactorSolar2 [order 2] : [after(KTHC_SolarDebounceT_sec*10,tick)]
  FactorSolar2.High -> FactorSolar1 [order 1] : [after(KTHC_SolarDebounceT_sec*10,tick)]
  (junction 11) -> FactorSolar2 [order 1] : [Solar>800]
  (junction 11) -> (junction 14) [order 2]
  FactorSolar2.Low -> FactorSolar3 [order 2] : [after(KTHC_SolarDebounceT_sec*10,tick)]
  FactorSolar3.High -> FactorSolar2 [order 2] : [after(KTHC_SolarDebounceT_sec*10,tick)]
  (junction 14) -> FactorSolar3 [order 1] : [Solar>650]
  (junction 14) -> (junction 17) [order 2]
  FactorSolar3.Low -> FactorSolar4.Low [order 2] : [after(KTHC_SolarDebounceT_sec*10,tick)]
  FactorSolar4.High -> FactorSolar3 [order 2] : [after(KTHC_SolarDebounceT_sec*10,tick)]
  (junction 17) -> FactorSolar4 [order 1] : [Solar>500]
  (junction 17) -> (junction 20) [order 2]
  FactorSolar4.Low -> FactorSolar5.Low [order 2] : [after(KTHC_SolarDebounceT_sec*10,tick)]
  FactorSolar5.High -> FactorSolar4 [order 2] : [after(KTHC_SolarDebounceT_sec*10,tick)]
  (junction 20) -> FactorSolar5 [order 1] : [Solar>350]
  (junction 20) -> (junction 23) [order 2]
  FactorSolar5.Low -> FactorSolar6.Low [order 2] : [after(KTHC_SolarDebounceT_sec*10,tick)]
  FactorSolar6.High -> FactorSolar5 [order 2] : [after(KTHC_SolarDebounceT_sec*10,tick)]
  (junction 23) -> FactorSolar6 [order 1] : [Solar>200]
  (junction 23) -> (junction 26) [order 2]
  FactorSolar7.High -> FactorSolar6 [order 2] : [after(KTHC_SolarDebounceT_sec*10,tick)]
  (junction 26) -> FactorSolar7
  data: Solar input; FactorSolar output single; KTHC_SolarDebounceT_sec input; Blowersolar output

== stateflow chart thc/THC/ThermalControl/THCM_Conctrl/BlowerCtrl/SlowIncrease ==
  state OFF
    en:Bout=0;
  state ON
    state Increase
      en:Bout=KTHC_VBstep_K;
      du:Bout=Bout+KTHC_VBstep_K;
    state Operating
      en:Bout=Bin;
      du:Bout=Bin;
    Increase -> Operating : [Bin<Bout+KTHC_VBstep_K]
  (default) -> OFF
  OFF -> Increase : [Bin>0]
  ON -> OFF : [Bin<=0]
  data: Bin input; Bout output; KTHC_VBstep_K input

== stateflow chart thc/THC/ThermalControl/THCM_Conctrl/Chart ==
  state CabinModeDet [parallel]
    settings: executionOrder=1
    state CabinMode4or5
    state Heating
    state Else
    (default) -> (junction 50)
    (junction 50) -> CabinMode4or5 [order 1] : [CabinMode==4||CabinMode==5]
    (junction 50) -> (junction 54) [order 2]
    CabinMode4or5 -> Heating [order 1] : [CabinMode==8||CabinMode==9]
        | {Balance=true;}
    (junction 65) -> CabinMode4or5 : [CabinMode==4||....
        | CabinMode==5]
    CabinMode4or5 -> Else [order 2] : [CabinMode!=4&&....
        | CabinMode!=5]
    Heating -> (junction 65) [order 1]
    (junction 54) -> Heating [order 1] : [CabinMode==8||CabinMode==9]
    (junction 54) -> Else [order 2]
    Else -> (junction 65) [order 2]
    Else -> Heating [order 1] : [CabinMode==8||CabinMode==9]
    Heating -> Else [order 2] : [CabinMode!=8&&....
        | CabinMode!=9]
  state HighPBalance [parallel]
    settings: executionOrder=2
    state DeCrease
      en:CompOut=CompOut-Step;
      du:CompOut=CompOut-Step;
    state Finish
      en:CompOut=CompIn;
      SOTXVout=SOTXV;
      du:CompOut=CompIn;
      SOTXVout=SOTXV;
    (default) -> (junction 9)
    HighPBalance -> (junction 9) : [Balance]{Balance=false;}
    (junction 9) -> DeCrease [order 1] : [CompOut>KTHC_CompSotxvOpLow_rpm&&....
        | PT_High_P>KTHC_SotxvProHi_kPa]....
        | {Step=(CompOut-KTHC_CompSotxvOpLow_rpm)/KTHC_CompSotxvOp_K;}
    (junction 9) -> (junction 14) [order 2]
    DeCrease -> Finish : [CompOut<KTHC_CompSotxvOpLow_rpm&&....
        | PT_High_P<KTHC_SotxvProLo_kPa]
    (junction 14) -> Finish
  data: CabinMode input; CompIn input; Step local double; CompOut output =0; SOTXVout output boolean =false; KTHC_CompSotxvOpLow_rpm input; KTHC_CompSotxvOp_K input; KTHC_SotxvProHi_kPa input; KTHC_SotxvProLo_kPa input; PT_High_P input; Balance local boolean; SOTXV input
